simulink model "motorslx"  (R2017b)
settings: Solver=VariableStepAuto  StartTime=0.0  StopTime=10.0  RelTol=1e-3
settings Model: Creator=Asus  LastModifiedBy=Asus

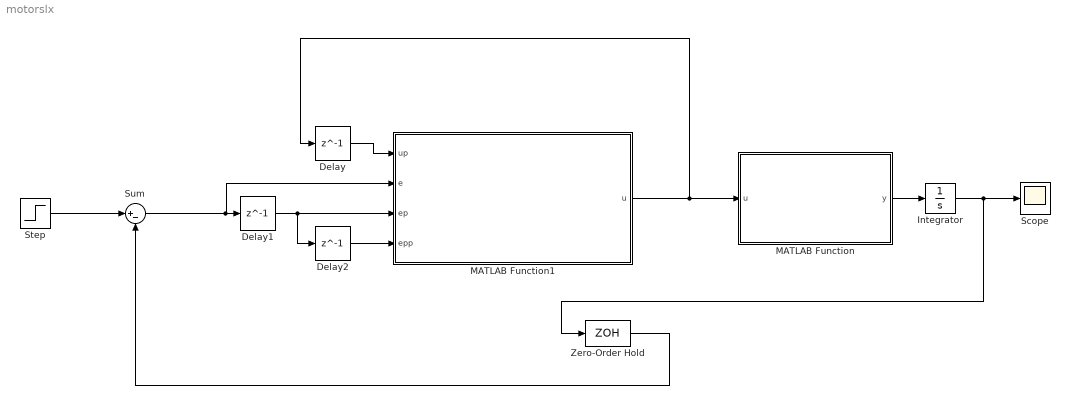
== system motorslx ==
  Delay : Delay  DelayLength=1  InitialCondition=0
  Delay1 : Delay  DelayLength=1  InitialCondition=0
  Delay2 : Delay  DelayLength=1  InitialCondition=0
  Integrator : Integrator
  MATLAB Function : MATLAB Function  TreatAsAtomicUnit=on
  MATLAB Function1 : MATLAB Function  TreatAsAtomicUnit=on
  Scope : Scope
  Step : Step  SampleTime=0
  Sum : Sum  Inputs=|+-
  Zero-Order Hold : ZeroOrderHold  SampleTime=-1
  wires:
  MATLAB Function1/1(u) -> Delay/1, MATLAB Function/1(u)
  Delay/1 -> MATLAB Function1/1(up)
  Delay1/1 -> Delay2/1, MATLAB Function1/3(ep)
  Delay2/1 -> MATLAB Function1/4(epp)
  MATLAB Function/1(y) -> Integrator/1
  Integrator/1 -> Zero-Order Hold/1, Scope/1
  Zero-Order Hold/1 -> Sum/2
  Step/1 -> Sum/1
  Sum/1 -> Delay1/1, MATLAB Function1/2(e)

== matlab function motorslx/MATLAB Function1 ==
  data: up input; u output; e input; ep input; epp input
function u = fcn(up,e,ep,epp)

Kp = 4.85;
Ki = 0.32;
Kd = 0;
Ts = 0.002;

u=  up+ (Kp+Ki*Ts/2+Kd/Ts)*e + (-Kp+Ki*Ts/2-2*Kd/Ts)*ep + (Kd/Ts)*epp;

== matlab function motorslx/MATLAB Function ==
  data: y output; u input
function y = motore(u)
Km = 1,08;
y = Km*u;
